simulink model "simulink_model"  (R2021b)
settings: Solver=VariableStepAuto  StartTime=0.0  StopTime=1000  RelTol=1e-3
InitFcn:
  | r=1/8;
  | u=0;
  | a=0.006;
  | b=0.1;
  | v=0;
  | e=1/3;
settings Model: Creator=Tisso  LastModifiedBy=Tisso

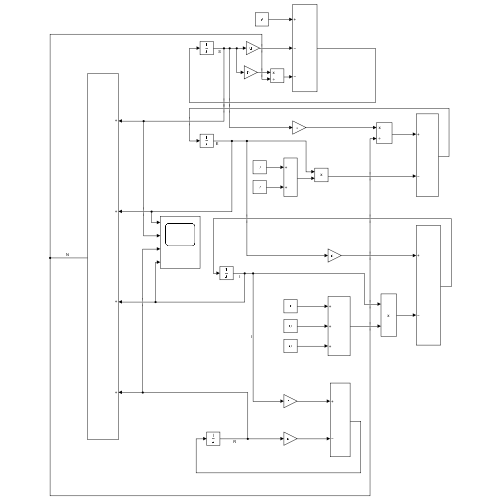
[thumbnail: Simulink's stored preview of the top-level diagram]
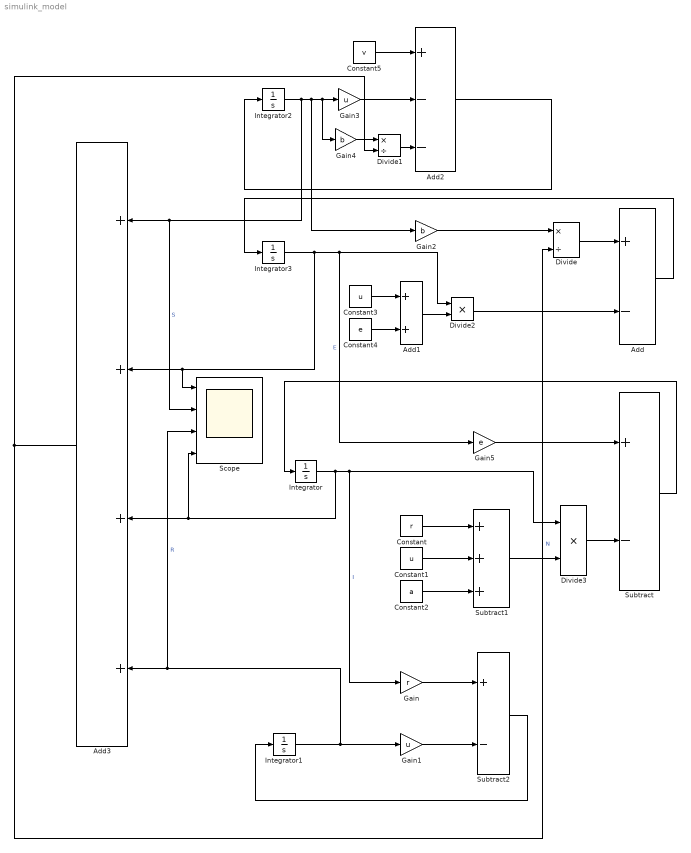
== system simulink_model ==
  Add : Sum  Inputs=+-
  Add1 : Sum
  Add2 : Sum  Inputs=+--
  Add3 : Sum  Inputs=++++
  Constant : Constant  Value=r
  Constant1 : Constant  Value=u
  Constant2 : Constant  Value=a
  Constant3 : Constant  Value=u
  Constant4 : Constant  Value=e
  Constant5 : Constant  Value=v
  Divide : Product  Inputs=*/
  Divide1 : Product  Inputs=*/
  Divide2 : Product  Inputs=**
  Divide3 : Product  Inputs=**
  Gain : Gain  Gain=r
  Gain1 : Gain  Gain=u
  Gain2 : Gain  Gain=b
  Gain3 : Gain  Gain=u
  Gain4 : Gain  Gain=b
  Gain5 : Gain  Gain=e
  Integrator : Integrator
  Integrator1 : Integrator
  Integrator2 : Integrator  InitialCondition=10
  Integrator3 : Integrator
  Scope : Scope  NumInputPorts=4
  Subtract : Sum  Inputs=+-
  Subtract1 : Sum  Inputs=+++
  Subtract2 : Sum  Inputs=+-
  wires:
  Subtract/1 -> Integrator/1
  Subtract2/1 -> Integrator1/1
  Constant2/1 -> Subtract1/3
  Constant1/1 -> Subtract1/2
  Constant/1 -> Subtract1/1
  Subtract1/1 -> Divide3/2
  Integrator/1 -> Scope/4, Add3/3, Gain/1, Divide3/1  "I"
  Divide3/1 -> Subtract/2
  Integrator1/1 -> Gain1/1, Scope/3, Add3/4  "R"
  Gain/1 -> Subtract2/1
  Gain1/1 -> Subtract2/2
  Constant4/1 -> Add1/2
  Constant3/1 -> Add1/1
  Add/1 -> Integrator3/1
  Constant5/1 -> Add2/1
  Integrator2/1 -> Scope/2, Add3/1, Gain2/1, Gain4/1, Gain3/1  "S"
  Gain3/1 -> Add2/2
  Add2/1 -> Integrator2/1
  Gain2/1 -> Divide/1
  Add3/1 -> Divide1/2, Divide/2  "N"
  Divide/1 -> Add/1
  Gain4/1 -> Divide1/1
  Divide1/1 -> Add2/3
  Gain5/1 -> Subtract/1
  Add1/1 -> Divide2/2
  Divide2/1 -> Add/2
  Integrator3/1 -> Scope/1, Add3/2, Divide2/1, Gain5/1  "E"
